simulink model "simulink_tirocinio4"  (R2021a)
settings: Solver=VariableStepAuto  StartTime=0.0  StopTime=100  RelTol=1e-3
values from neighbouring files (symbols this model uses):
  A_n = [0 0 1 0; 0 0 0 1; -k/m1 k/m1 -c/m1 c/m1; k/m2 -k/m2 c/m2 -c/m2]    [tirocinio3_complessiconiugati.m]    (also in tirocinio3_immaginari_puri.m; tirocinio3_reali.m; tirocinio4_rampa.m; tirocinio4_sinusoide.m)
  Ac = A_segn - V*C_segn + B_segn*F - V*D_segn*F    [tirocinio4_rampa.m]    (also in tirocinio4_sinusoide.m = [As zeros(6, 2); Bm*Cs Am])
  B_n = [0; 0; 1/m1; 0]    [tirocinio3_complessiconiugati.m]    (also in tirocinio3_immaginari_puri.m; tirocinio3_reali.m; tirocinio4_rampa.m; tirocinio4_sinusoide.m)
  Bc = V    [tirocinio4_rampa.m]    (also in tirocinio4_sinusoide.m = [Bs; Bm*Ds])
  C_n = [1 0 0 0]    [tirocinio3_complessiconiugati.m]    (also in tirocinio3_immaginari_puri.m; tirocinio3_reali.m; tirocinio4_rampa.m; tirocinio4_sinusoide.m)
  Cc = -F    [tirocinio4_rampa.m]    (also in tirocinio4_sinusoide.m = [Dm*Cs Cm])
  D_n = 0    [tirocinio3_complessiconiugati.m]    (also in tirocinio3_immaginari_puri.m; tirocinio3_reali.m; tirocinio4_rampa.m; tirocinio4_sinusoide.m)
  Dc = 0    [tirocinio4_rampa.m]    (also in tirocinio4_sinusoide.m)
  M = [0; 0; 0; 1/m2_m]    [tirocinio3_complessiconiugati.m]    (also in tirocinio3_immaginari_puri.m; tirocinio3_reali.m; tirocinio4_rampa.m = 2; tirocinio4_sinusoide.m = 1)
  M0 = 2    [tirocinio4_rampa.m]    (also in tirocinio4_sinusoide.m = 1)
  M1 = 1    [tirocinio4_rampa.m]    (also in tirocinio4_sinusoide.m)
  phi = pi/2    (= 1.57079632679)    [tirocinio4_rampa.m]    (also in tirocinio4_sinusoide.m = 2)
  w = 1    [tirocinio4_rampa.m]    (also in tirocinio4_sinusoide.m)
  x0 = [0;2;0;0]    [tirocinio3_complessiconiugati.m]    (also in tirocinio3_immaginari_puri.m; tirocinio3_reali.m = [1;10;3;2]; tirocinio4_rampa.m = [0; 2; 0; 0]; tirocinio4_sinusoide.m = [0;0;0;0])
libraries: simulink x1
settings Model: Creator=Valentina  LastModifiedBy=Valentina

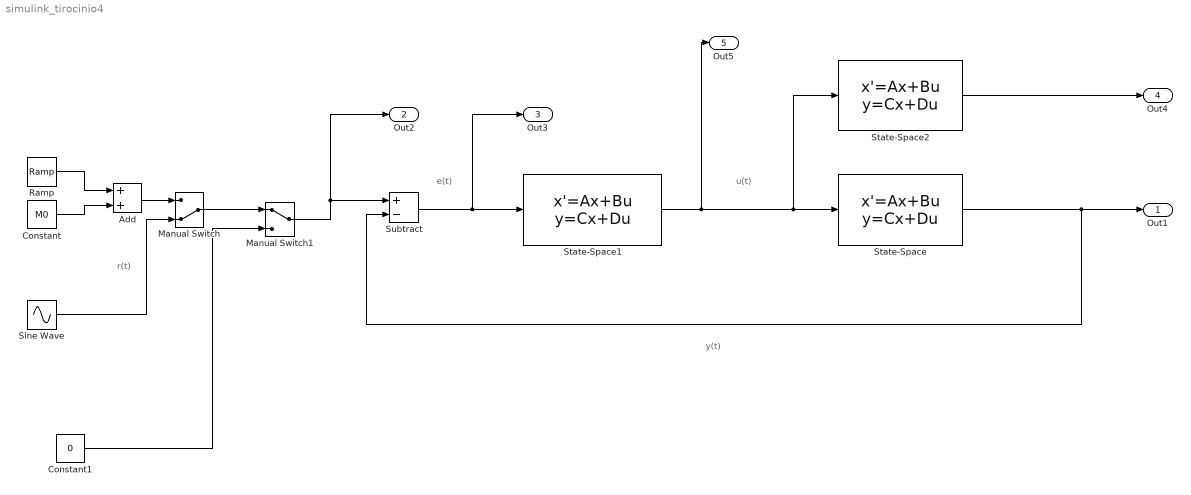
== system simulink_tirocinio4 ==
  note: y(t)
  note: r(t)
  note: u(t)
  note: e(t)
  Add : Sum
  Constant : Constant  Value=M0
  Constant1 : Constant  Value=0
  Manual Switch : ManualSwitch  CurrentSetting=0
  Manual Switch1 : ManualSwitch
  Ramp : simulink/Sources/Ramp  slope=M1  start=0  InitialOutput=0
  Sine Wave : Sin  Amplitude=M  Frequency=w  Phase=phi  SampleTime=0
  State-Space : StateSpace  A=A_n  B=B_n  C=C_n  D=D_n  InitialCondition=x0
  State-Space1 : StateSpace  A=Ac  B=Bc  C=Cc  D=Dc  InitialCondition=0
  State-Space2 : StateSpace  A=A_n  B=B_n  C=eye(4)  D=[0;0;0;0]  InitialCondition=x0
  Subtract : Sum  Inputs=+-
  Out1 : Outport  SignalName=y(t)
  Out2 : Outport  Port=2  SignalName=r(t)
  Out3 : Outport  Port=3  SignalName=e(t)
  Out4 : Outport  Port=4  SignalName=x(t)
  Out5 : Outport  Port=5
  wires:
  State-Space1/1 -> Out5/1, State-Space2/1, State-Space/1
  State-Space/1 -> Subtract/2, Out1/1
  Subtract/1 -> Out3/1, State-Space1/1
  Ramp/1 -> Add/1
  Constant/1 -> Add/2
  Add/1 -> Manual Switch/1
  Sine Wave/1 -> Manual Switch/2
  State-Space2/1 -> Out4/1
  Manual Switch1/1 -> Out2/1, Subtract/1
  Manual Switch/1 -> Manual Switch1/1
  Constant1/1 -> Manual Switch1/2
